simulink model "schemaacfir"  (R2017b)
settings: Solver=FixedStepAuto  StartTime=0.0  StopTime=0.1  FixedStep=1/4000  MaxStep=1/4000  RelTol=1e-3
libraries: dspsrcs4 x1, dsparch4 x1, fillib x1
settings Model: Creator=test  LastModifiedBy=test

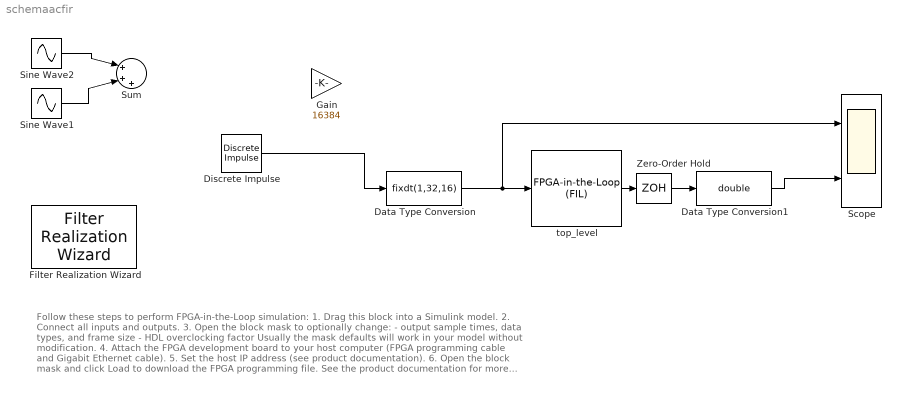
== system schemaacfir ==
  note: Follow these steps to perform FPGA-in-the-Loop simulation:
      |
      | 1. Drag this block into a Simulink model.
      | 2. Connect all inputs and outputs.
      | 3. Open the block mask to optionally change:
      |     - output sample times, data types, and frame size
      |     - HDL overclocking factor
      |     Usually the mask defaults will work in your model without modification.
      | 4. Attach the FPGA development board to your host computer (FPGA
      |     programming cable and Gigabit Ethernet cable).
      | 5. Set the host IP address (see product documentation).
      | 6. Open the block mask and click Load to download the FPGA programming file.
      |
      | See the product documentation for more detailed instructions and
      | troubleshooting tips.
  Data Type Conversion : DataTypeConversion  OutDataTypeStr=fixdt(1,32,16)
  Data Type Conversion1 : DataTypeConversion  OutDataTypeStr=double
  Discrete Impulse : dspsrcs4/Discrete  Impulse  Delay=100  SampleTime=25e-5  FrameSample=1  OutputFrames=off  dataType=single  isSigned=on  wordLen=32  udDataType=sfix(16)  fracBitsMode=User-defined  numFracBits=16  OutDataTypeStr=single  LastOutDataTypeStr=single
  Filter Realization Wizard : dsparch4/Filter Realization Wizard
      settings: SourceProductName=DSP System Toolbox  SourceProductBaseCode=DS
  Gain : Gain  Gain=16384  OutDataTypeStr=double
  Scope : Scope  NumInputPorts=2
  Sine Wave1 : Sin  Amplitude=50  Frequency=500  SampleTime=25e-5
  Sine Wave2 : Sin  Amplitude=50  Frequency=1000  SampleTime=25e-5
  Sum : Sum  Inputs=|+++
  Zero-Order Hold : ZeroOrderHold  SampleTime=1/4000
  top_level : fillib/FPGA-in-the-Loop (FIL)  ForceInterfaceUpdate=0.90579
  wires:
  Sine Wave1/1 -> Sum/2
  Sine Wave2/1 -> Sum/1
  top_level/1 -> Zero-Order Hold/1
  Zero-Order Hold/1 -> Data Type Conversion1/1
  Discrete Impulse/1 -> Data Type Conversion/1
  Data Type Conversion/1 -> Scope/1, top_level/1
  Data Type Conversion1/1 -> Scope/2
